simulink model "q3"  (R2018b)
settings: Solver=FixedStepDiscrete  StartTime=0.0  StopTime=10000  FixedStep=0.5  RelTol=1e-3  EnableMultiTasking=on
libraries: simulink_extras x1
settings Model: PauseTimes=120  SnapshotInterval=4  Creator=lenovo  LastModifiedBy=lenovo
settings SolverCC: AutoInsertRateTranBlk=on
settings DataIOCC: ExternalInput=[t, a, b, c, d, e, f, g]  LimitDataPoints=on
settings OptimizationCC: LifeSpan=inf
settings DebuggingCC: AllowSymbolicDim=off  SFUnexpectedBacktrackingDiag=warning  SFNoUnconditionalDefaultTransitionDiag=warning  SFExecutionAtInitializationDiag=none
settings SFSimCC: SimUseLocalCustomCode=off
settings RTWCC: RTWUseLocalCustomCode=off
settings CodeAppCC: StateflowObjectComments=on
settings GRTTargetCC: TargetLangStandard=C89/C90 (ANSI)  GeneratePreprocessorConditionals=Disable all
settings ConfigComp: CovMetricSettings=dw  CovHtmlReporting=on  CovSaveCumulativeToWorkspaceVar=on  CovSaveSingleToWorkspaceVar=on  CovShowResultsExplorer=off  CovExternalEMLEnable=off  CovSFcnEnable=off

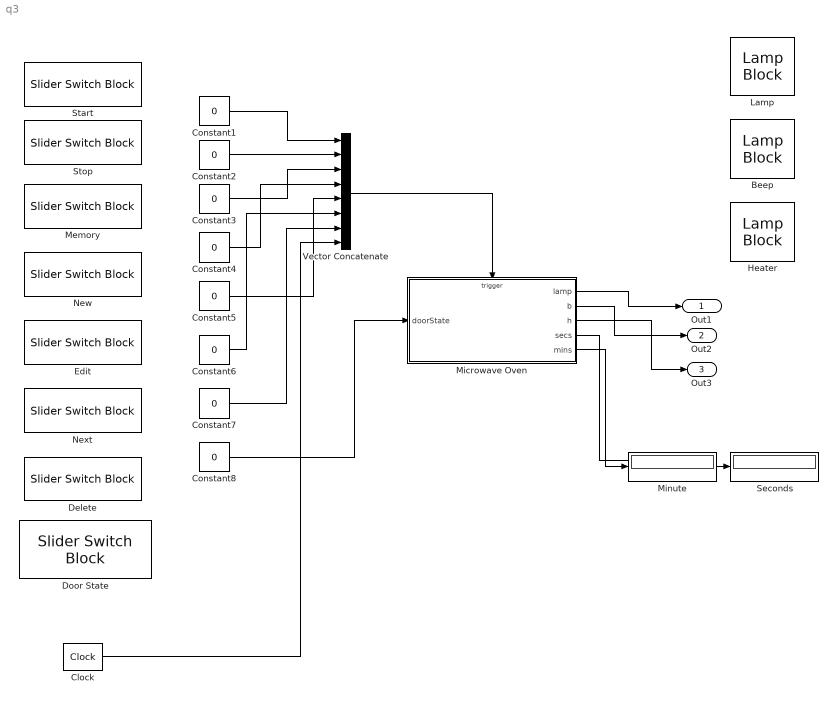
== system q3 ==
  Beep : LampBlock  WebBlockId=59  LabelPosition=Hide
  Clock : simulink_extras/Flip Flops/Clock  period=2
  Constant{1..7} (7 alike) : Constant  Value=0
  Constant8 : Constant  Value=0  OutDataTypeStr=boolean
  Delete : SliderSwitchBlock  WebBlockId=55  LabelPosition=Hide
      settings: Values={{'Off', 'On'}, [0 1]}
  Door State : SliderSwitchBlock  WebBlockId=25  LabelPosition=Hide
      settings: Values={{'Closed', 'Opened'}, [0 1]}
  "Edit " : SliderSwitchBlock  WebBlockId=52  LabelPosition=Hide
      settings: Values={{'Off', 'On'}, [0 1]}
  Heater : LampBlock  WebBlockId=60  LabelPosition=Hide
  Lamp : LampBlock  WebBlockId=58  LabelPosition=Hide
  Memory : SliderSwitchBlock  WebBlockId=50  LabelPosition=Hide
      settings: Values={{'Off', 'On'}, [0 1]}
  Microwave Oven : Stateflow chart  TreatAsAtomicUnit=on
  Minute : Display
  New : SliderSwitchBlock  WebBlockId=51  LabelPosition=Hide
      settings: Values={{'Off', 'On'}, [0 1]}
  Next : SliderSwitchBlock  WebBlockId=53  LabelPosition=Hide
      settings: Values={{'Off', 'On'}, [0 1]}
  Seconds : Display
  Start : SliderSwitchBlock  WebBlockId=48  LabelPosition=Hide
      settings: Values={{'Off', 'On'}, [0 1]}
  Stop : SliderSwitchBlock  WebBlockId=49  LabelPosition=Hide
      settings: Values={{'Off', 'On'}, [0 1]}
  Vector Concatenate : Concatenate  NumInputs=8
  Out1 : Outport
  Out2 : Outport  Port=2
  Out3 : Outport  Port=3
  wires:
  Vector Concatenate/1 -> Microwave Oven/Trigger
  Constant1/1 -> Vector Concatenate/1
  Constant2/1 -> Vector Concatenate/2
  Constant3/1 -> Vector Concatenate/3
  Constant4/1 -> Vector Concatenate/4
  Constant5/1 -> Vector Concatenate/5
  Constant6/1 -> Vector Concatenate/6
  Constant7/1 -> Vector Concatenate/7
  Microwave Oven/5(mins) -> Minute/1
  Microwave Oven/4(secs) -> Seconds/1
  Microwave Oven/1(lamp) -> Out1/1
  Microwave Oven/2(b) -> Out2/1
  Microwave Oven/3(h) -> Out3/1
  Clock/1 -> Vector Concatenate/8
  Constant8/1 -> Microwave Oven/1(doorState)

== stateflow chart q3/Microwave Oven ==
  state display_subsystem [parallel]
    settings: executionOrder=4
    state time
      entry: mins = cookingTime/60
      secs = cookingTime %% 60
    state savedTime
      entry: mins = savedTimes[savedTimeIdx] / 60
      secs = savedTimes[savedTimeIdx] %% 60
    state error
      entry: mins=-1
      secs=-1
    (default) -> time
    time -> savedTime [order 1] : [displaySavedTime==1 && displayTime==0 && displayError==0]
    savedTime -> time [order 1] : [displaySavedTime==0 && displayTime==1 && displayError==0]
    time -> display_subsystem.error [order 2] : [displaySavedTime==0 && displayTime==0 && displayError==1]
    savedTime -> display_subsystem.error [order 2] : [displaySavedTime==0 && displayTime==0 && displayError==1]
    time -> time [order 3] : after(500, msec)
    display_subsystem.error -> time [order 1] : [displaySavedTime==0 && displayTime==1 && displayError==0]
    display_subsystem.error -> savedTime [order 2] : [displaySavedTime==1 && displayTime==0 && displayError==0]
    savedTime -> savedTime [order 3] : after(500, msec)
  state beep_subsystem [parallel]
    settings: executionOrder=3
    state ON
      entry: b = beep(1)
    state OFF
      entry: b=beep(0)
    (default) -> beep_subsystem.OFF
    beep_subsystem.ON -> beep_subsystem.OFF : [beep==0]
    beep_subsystem.OFF -> beep_subsystem.ON : [beep==1]
  state light_subsystem [parallel]
    settings: executionOrder=2
    state OFF
      entry:
      lamp=lightOff()
    state ON
      entry:
      lamp=lightOn()
    (default) -> light_subsystem.OFF
    light_subsystem.ON -> light_subsystem.OFF : [light==0 && doorState==0]
    light_subsystem.OFF -> light_subsystem.ON : [light==1 || doorState==1]
  state heating_subsystem [parallel]
    settings: executionOrder=5
    state OFF
      entry:
      h = heaterOff()
    state ON
      entry:
      h = heaterOn()
    (default) -> heating_subsystem.OFF
    heating_subsystem.OFF -> heating_subsystem.ON : [heater==1]
    heating_subsystem.ON -> heating_subsystem.OFF : [heater==0]
  state control_subsystem [parallel]
    settings: executionOrder=1
    state edit_sec
    state edit_min
    state memory
      entry: displayTime = 0
      entry: displayError = 0
      entry: displaySavedTime = 1
    state beeping
      entry: beep = 1
      on timerClock:
      beepTime = beepTime - 1
      exit: beep = 0
    state idle
      entry: cookingTime = 0
      entry: displayTime = 1
      entry: displaySavedTime = 0
      entry: beepTime = 0
      entry: displayError = 0
    state cooking
      entry: light = 1
      entry: heater = 1
      on startButtonPushed:
      cookingTime = cookingTime + 30
      on timerClock:
      cookingTime = cookingTime - 1
      exit: heater = 0
      light = 0
    state error
      entry: displayTime = 0
      entry: displayError = 1
      entry: displaySavedTime = 0
    state pause
    edit_sec -> memory [order 2] : editButtonPushed
    edit_sec -> edit_sec [order 1] : nextButtonPushed{savedTimes[savedTimeIdx]=savedTimes[savedTimeIdx]+1}
    edit_min -> edit_sec [order 2] : editButtonPushed
    memory -> edit_min [order 5] : newButtonPushed{numberOfSavedTimes=numberOfSavedTimes+1, savedTimeIdx=numberOfSavedTimes-1}
    edit_min -> edit_min [order 1] : nextButtonPushed{savedTimes[savedTimeIdx]=savedTimes[savedTimeIdx]+60}
    memory -> edit_min [order 4] : editButtonPushed
    control_subsystem.error -> edit_min [order 1] : newButtonPushed{numberOfSavedTimes=numberOfSavedTimes+1, savedTimeIdx=numberOfSavedTimes-1, displaySavedTime = 1, displayError = 0}
    memory -> control_subsystem.error [order 7] : deleteButtonPushed[savedTimeIdx >= (numberOfSavedTimes-1) && numberOfSavedTimes <= 1]{numberOfSavedTimes = numberOfSavedTimes-1, savedTimes=deleteSavedTime(savedTimes, savedTimeIdx)}
    memory -> memory [order 2] : nextButtonPushed{savedTimeIdx = (savedTimeIdx+1)%%numberOfSavedTimes}
    memory -> memory [order 1] : deleteButtonPushed[savedTimeIdx < (numberOfSavedTimes-1)]{savedTimes=deleteSavedTime(savedTimes, savedTimeIdx), numberOfSavedTimes=numberOfSavedTimes-1}
    beeping -> idle [order 3] : [beepTime==0]
    beeping -> idle [order 2] : [doorState==1]
    memory -> cooking [order 3] : startButtonPushed[doorState==0]{cookingTime=savedTimes[savedTimeIdx], displayTime=1, displaySavedTime=0, displayError=0}
    memory -> memory [order 6] : deleteButtonPushed[savedTimeIdx >= (numberOfSavedTimes-1) && numberOfSavedTimes > 1]{numberOfSavedTimes = numberOfSavedTimes-1,  savedTimes=deleteSavedTime(savedTimes, savedTimeIdx)}
    memory -> idle [order 8] : memoryButtonPushed
    idle -> memory [order 2] : memoryButtonPushed[numberOfSavedTimes > 0]{savedTimeIdx=0}
    beeping -> cooking [order 1] : startButtonPushed[doorState==0]{cookingTime = cookingTime + 30}
    cooking -> beeping [order 3] : [cookingTime==0]{beepTime = 3}
    (default) -> idle
    idle -> cooking [order 1] : startButtonPushed[doorState==0]{cookingTime = cookingTime + 30}
    cooking -> pause [order 1] : stopButtonPushed
    cooking -> pause [order 2] : [doorState==1]
    pause -> cooking [order 1] : startButtonPushed[doorState==0]
    control_subsystem.error -> idle [order 2] : memoryButtonPushed
    idle -> control_subsystem.error [order 3] : memoryButtonPushed[numberOfSavedTimes==0]
    pause -> idle [order 2] : stopButtonPushed
  data: s function_input double; answer function_output double; answer function_output double; answer function_output double; answer function_output double; answer function_output double; array function_input double size=[1 10]; idx function_input double size=1; newSavedTimes function_output double size=[1 10]; cookingTime local int32 size=1 =0; beepTime local int32 size=1 =0; displayTime local boolean size=1 =1; displaySavedTime local boolean size=1 =0; savedTimes local int32 size=[1 10]; savedTimeIdx local int32 size=1 =0; numberOfSavedTimes local int32 size=1 =0; light local boolean size=1 =0; displayError local boolean size=1 =0; beep local boolean size=1 =0; doorState input boolean size=1; heater local boolean size=1 =0; lamp output double; b output double; h output double; secs output double; mins output double
  events: startButtonPushed input RISING_EDGE_EVENT; stopButtonPushed input RISING_EDGE_EVENT; memoryButtonPushed input RISING_EDGE_EVENT; newButtonPushed input RISING_EDGE_EVENT; editButtonPushed input RISING_EDGE_EVENT; nextButtonPushed input RISING_EDGE_EVENT; deleteButtonPushed input RISING_EDGE_EVENT; timerClock input EITHER_EDGE_EVENT
  function answer = beep(s):
    | function answer = beep(s)
    |     answer = s;
    | end
  function answer = lightOn:
    | function answer = lightOn
    |     answer = 1;
    | end
  function answer = lightOff:
    | function answer = lightOff
    |     answer = 0;
    | end
  function answer = heaterOn:
    | function answer = heaterOn
    |     answer = 1;
    | end
  function answer = heaterOff:
    | function answer = heaterOff
    |     answer = 0;
    | end
  function newSavedTimes = deleteSavedTime(array, idx):
    | function newSavedTimes = deleteSavedTime(array, idx)
    |     
    |     idx = idx+1;
    |     newSavedTimes = array(:, :);
    |     n = length(array);
    |     for i=idx:n-1
    |         newSavedTimes(1, i) = newSavedTimes(1, i+1);
    |     end
    |     newSavedTimes(1, n) = 0;
    | end
